simulink model "steer_to_rwa_in"  (R2023b)
settings: Solver=VariableStepAuto  StartTime=0.0  StopTime=20  RelTol=1e-3
model workspace (MAT data in the model file):
  x = 4
libraries: simulink x3
settings Model: Creator=jcm52  LastModifiedBy=jcm52

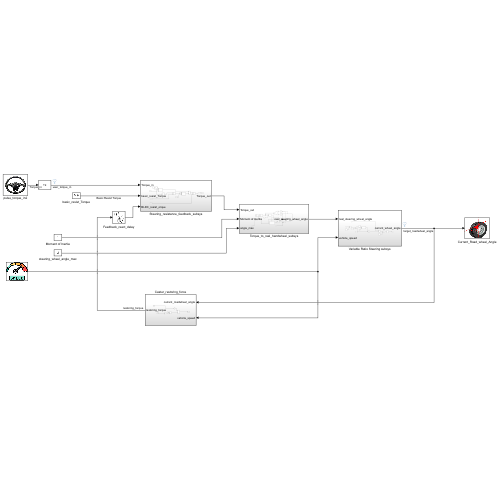
[thumbnail: Simulink's stored preview of the top-level diagram]
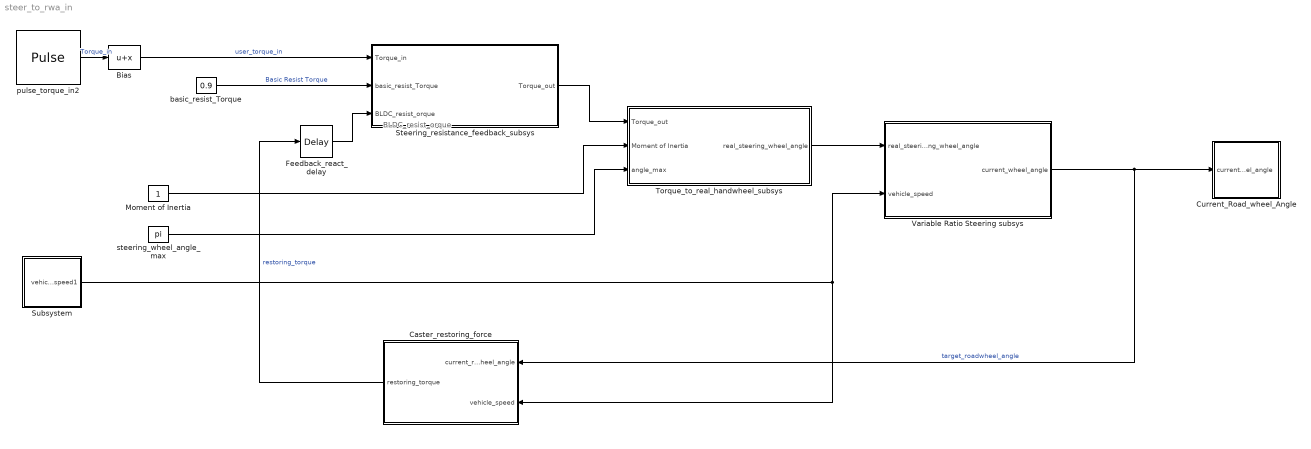
== system steer_to_rwa_in ==
  note: BLDC_resist_orque
  Bias : Bias  Bias=x  SaturateOnIntegerOverflow=off
  Caster_restoring_force : Subsystem
  Current_Road_wheel_Angle : Subsystem
      mask Display: image('image\road_wheel_angle.JPG');
  Feedback_react_delay : TransportDelay  DelayTime=0.02
  Moment of Inertia : Constant
  Steering_resistance_feedback_subsys : Subsystem
  Subsystem : Subsystem
      mask Display: image('image\free-icon-speed-1455318.png');
  Torque_to_real_handwheel_subsys : Subsystem
  Variable Ratio Steering subsys : Subsystem
  basic_resist_Torque : Constant  Value=0.9  SampleTime=0.001
  pulse_torque_in2 : DiscretePulseGenerator  PulseType=Time based  Amplitude=2*x  Period=5  PulseWidth=50
      mask Display: image('image\pngtree-car-steering-wheel-png-image_13061877.png');
  steering_wheel_angle_max : Constant  Value=pi
  wires:
  Bias/1 -> Steering_resistance_feedback_subsys/1(Torque_in)  "user_torque_in"
  basic_resist_Torque/1 -> Steering_resistance_feedback_subsys/2(basic_resist_Torque)  "Basic Resist Torque"
  Feedback_react_delay/1 -> Steering_resistance_feedback_subsys/3(BLDC_resist_orque)
  Steering_resistance_feedback_subsys/1(Torque_out) -> Torque_to_real_handwheel_subsys/1(Torque_out)
  Moment of Inertia/1 -> Torque_to_real_handwheel_subsys/2(Moment of Inertia)
  steering_wheel_angle_max/1 -> Torque_to_real_handwheel_subsys/3(angle_max)
  Torque_to_real_handwheel_subsys/1(real_steering_wheel_angle) -> Variable Ratio Steering subsys/1(real_steering_wheel_angle)
  Variable Ratio Steering subsys/1(current_wheel_angle) -> Current_Road_wheel_Angle/1(current_wheel_angle), Caster_restoring_force/1(current_roadwheel_angle)  "target_roadwheel_angle"
  pulse_torque_in2/1 -> Bias/1  "Torque_in"
  Caster_restoring_force/1(restoring_torque) -> Feedback_react_delay/1  "restoring_torque"
  Subsystem/1(vehicle_speed1) -> Variable Ratio Steering subsys/2(vehicle_speed), Caster_restoring_force/2(vehicle_speed)

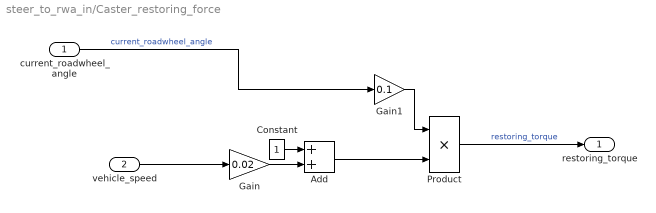
== system steer_to_rwa_in/Caster_restoring_force ==
  current_roadwheel_angle : Inport
  vehicle_speed : Inport  Port=2
  Add : Sum
  Constant : Constant
  Gain : Gain  Gain=0.02
  Gain1 : Gain  Gain=0.1
  Product : Product
  restoring_torque : Outport
  wires:
  vehicle_speed/1 -> Gain/1
  Gain/1 -> Add/2
  Constant/1 -> Add/1
  Add/1 -> Product/2
  Gain1/1 -> Product/1
  Product/1 -> restoring_torque/1  "restoring_torque"
  current_roadwheel_angle/1 -> Gain1/1  "current_roadwheel_angle"

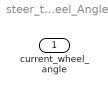
== system steer_to_rwa_in/Current_Road_wheel_Angle ==
  current_wheel_angle : Inport

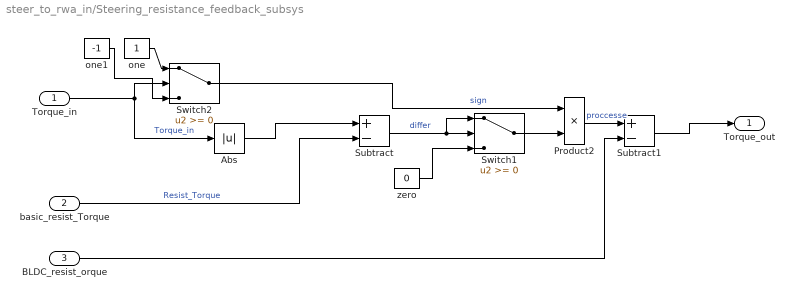
== system steer_to_rwa_in/Steering_resistance_feedback_subsys ==
  Torque_in : Inport
  basic_resist_Torque : Inport  Port=2
  BLDC_resist_orque : Inport  Port=3
  Abs : Abs  SaturateOnIntegerOverflow=off
  Product2 : Product
  Subtract : Sum  Inputs=+-
  Subtract1 : Sum  Inputs=+-
  Switch1 : Switch  OutDataTypeStr=double  SaturateOnIntegerOverflow=off  InputSameDT=off
  Switch2 : Switch  OutDataTypeStr=double  SaturateOnIntegerOverflow=off  InputSameDT=off
  one : Constant
  one1 : Constant  Value=-1
  zero : Constant  Value=0
  Torque_out : Outport
  wires:
  Subtract/1 -> Switch1/1, Switch1/2  "differ"
  one/1 -> Switch2/1
  basic_resist_Torque/1 -> Subtract/2  "Resist_Torque"
  zero/1 -> Switch1/3
  Torque_in/1 -> Switch2/2, Abs/1  "Torque_in"
  Switch1/1 -> Product2/2
  Switch2/1 -> Product2/1  "sign"
  Abs/1 -> Subtract/1
  one1/1 -> Switch2/3
  BLDC_resist_orque/1 -> Subtract1/2
  Product2/1 -> Subtract1/1  "proccesse"
  Subtract1/1 -> Torque_out/1

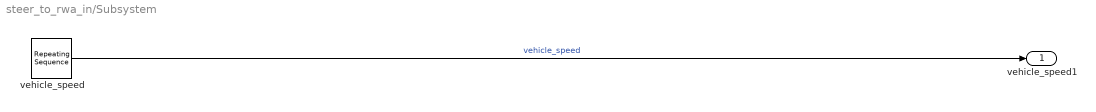
== system steer_to_rwa_in/Subsystem ==
  vehicle_speed : simulink/Sources/Repeating Sequence  rep_seq_t=[0 50 100]  rep_seq_y=[0 200 0]
  vehicle_speed1 : Outport
  wires:
  vehicle_speed/1 -> vehicle_speed1/1  "vehicle_speed"

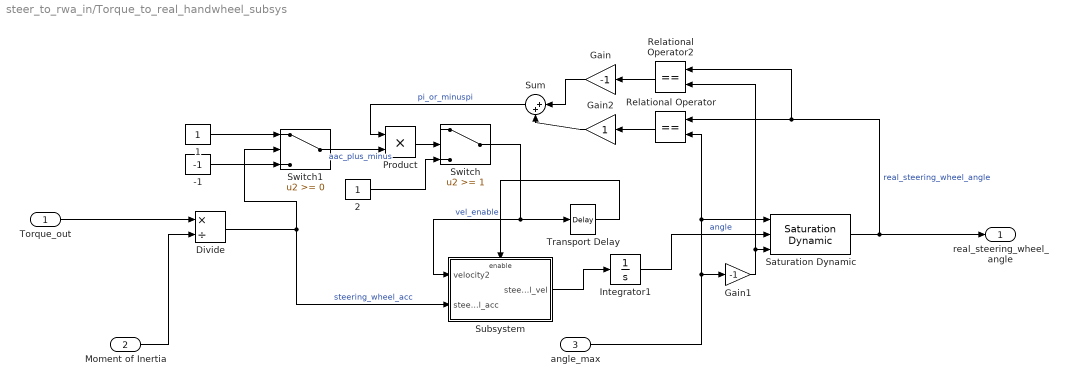
== system steer_to_rwa_in/Torque_to_real_handwheel_subsys ==
  Torque_out : Inport
  Moment of Inertia : Inport  Port=2
  angle_max : Inport  Port=3
  -1 : Constant  Value=-1
  1 : Constant
  2 : Constant  OutDataTypeStr=boolean
  Divide : Product  Inputs=*/
  Gain : Gain  Gain=-1
  Gain1 : Gain  Gain=-1
  Gain2 : Gain
  Integrator1 : Integrator
  Product : Product
  Relational Operator : RelationalOperator  Operator===  OutDataTypeStr=boolean  RndMeth=Simplest  InputSameDT=off
  Relational Operator2 : RelationalOperator  Operator===  OutDataTypeStr=boolean  RndMeth=Simplest  InputSameDT=off
  Saturation Dynamic : simulink/Discontinuities/Saturation Dynamic  OutMin=[]  OutMax=[]  OutDataTypeStr=double  OutDataType=fixdt(1, 16)  OutScaling=2^-10  DoSatur=off
  Subsystem : Subsystem
  Sum : Sum  Inputs=|++
  Switch : Switch  Threshold=1  OutDataTypeStr=double  SaturateOnIntegerOverflow=off  InputSameDT=off
  Switch1 : Switch  SaturateOnIntegerOverflow=off  InputSameDT=off
  Transport Delay : TransportDelay  DelayTime=0.001
  real_steering_wheel_angle : Outport
  wires:
  Saturation Dynamic/1 -> Relational Operator2/1, Relational Operator/1, real_steering_wheel_angle/1  "real_steering_wheel_angle"
  Torque_out/1 -> Divide/1
  Integrator1/1 -> Saturation Dynamic/2  "angle"
  angle_max/1 -> Relational Operator/2, Saturation Dynamic/1, Gain1/1
  Gain1/1 -> Relational Operator2/2, Saturation Dynamic/3
  Moment of Inertia/1 -> Divide/2
  Divide/1 -> Switch1/2, Subsystem/2(steering_wheel_acc)  "steering_wheel_acc"
  Subsystem/1(steering_wheel_vel) -> Integrator1/1
  Switch/1 -> Subsystem/1(velocity2), Transport Delay/1  "vel_enable"
  Sum/1 -> Product/1  "pi_or_minuspi"
  -1/1 -> Switch1/3
  1/1 -> Switch1/1
  Switch1/1 -> Product/2  "aac_plus_minus"
  Relational Operator2/1 -> Gain/1
  Relational Operator/1 -> Gain2/1
  Gain/1 -> Sum/1
  Product/1 -> Switch/2
  2/1 -> Switch/3
  Gain2/1 -> Sum/2
  Transport Delay/1 -> Subsystem/Enable

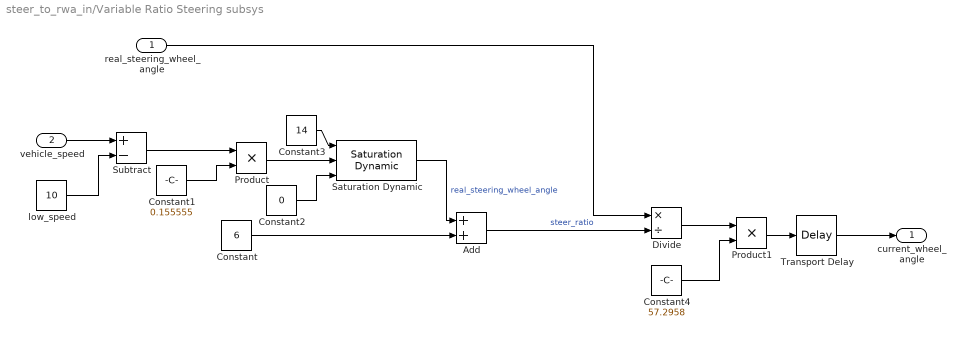
== system steer_to_rwa_in/Variable Ratio Steering subsys ==
  real_steering_wheel_angle : Inport
  vehicle_speed : Inport  Port=2
  Add : Sum
  Constant : Constant  Value=6
  Constant1 : Constant  Value=0.155555
  Constant2 : Constant  Value=0
  Constant3 : Constant  Value=14
  Constant4 : Constant  Value=57.2958
  Divide : Product  Inputs=*/
  Product : Product
  Product1 : Product
  Saturation Dynamic : simulink/Discontinuities/Saturation Dynamic  OutMin=[]  OutMax=[]  OutDataTypeStr=double  OutDataType=fixdt(1, 16)  OutScaling=2^-10  DoSatur=off
  Subtract : Sum  Inputs=+-
  Transport Delay : TransportDelay  DelayTime=0.1
  low_speed : Constant  Value=10
  current_wheel_angle : Outport
  wires:
  vehicle_speed/1 -> Subtract/1
  low_speed/1 -> Subtract/2
  Subtract/1 -> Product/1
  Constant1/1 -> Product/2
  Constant/1 -> Add/2
  Product/1 -> Saturation Dynamic/2
  Constant2/1 -> Saturation Dynamic/3
  Constant3/1 -> Saturation Dynamic/1
  Saturation Dynamic/1 -> Add/1  "real_steering_wheel_angle"
  Add/1 -> Divide/2  "steer_ratio"
  real_steering_wheel_angle/1 -> Divide/1
  Divide/1 -> Product1/1
  Constant4/1 -> Product1/2
  Product1/1 -> Transport Delay/1
  Transport Delay/1 -> current_wheel_angle/1

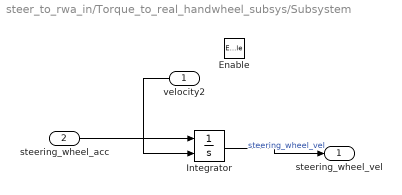
== system steer_to_rwa_in/Torque_to_real_handwheel_subsys/Subsystem ==
  velocity2 : Inport
  steering_wheel_acc : Inport  Port=2
  Enable : EnablePort  StatesWhenEnabling=reset
  Integrator : Integrator  ExternalReset=either
  steering_wheel_vel : Outport
  wires:
  Integrator/1 -> steering_wheel_vel/1  "steering_wheel_vel"
  velocity2/1 -> Integrator/2
  steering_wheel_acc/1 -> Integrator/1
